simulink model "vehicle_progetto_v1_sospensioni_dual_motor"  (R2022a)
settings: Solver=ode45  StartTime=0.0  StopTime=200.0  MinStep=1e-60  RelTol=1e-3
values from neighbouring files (symbols this model uses):
  a = 1.3    [vehicle_parameters_v1_sospensioni.m]
  alpha = atan(w/(2*b))    [vehicle_parameters_v1_sospensioni.m]
  b = 1.8    [vehicle_parameters_v1_sospensioni.m]
  ca = 0.5    [vehicle_parameters_v1_sospensioni.m]
  cs = sqrt(2*ks*M)    [vehicle_parameters_v1_sospensioni.m]
  h_gc = 0.35    [vehicle_parameters_v1_sospensioni.m]
  J_motore = 0.3    [vehicle_parameters_v1_sospensioni.m]
  J_wheel = 0.4    [vehicle_parameters_v1_sospensioni.m]
  Jx = 300    [vehicle_parameters_v1_sospensioni.m]
  Jy = 500    [vehicle_parameters_v1_sospensioni.m]
  Jz = 600    [vehicle_parameters_v1_sospensioni.m]
  K_elettrica_motore = 0.1    [vehicle_parameters_v1_sospensioni.m]
  K_f_motore = 1    [vehicle_parameters_v1_sospensioni.m]
  K_motore = 1    [vehicle_parameters_v1_sospensioni.m]
  k_r = 200*1e4    (= 2000000)    [vehicle_parameters_v1_sospensioni.m]
  k_tu = 10*1.5e5    (= 1500000)    [vehicle_parameters_v1_sospensioni.m]
  k_tv = 10*40000    (= 400000)    [vehicle_parameters_v1_sospensioni.m]
  ks = 39000/4    (= 9750)    [vehicle_parameters_v1_sospensioni.m]
  L = sqrt(a^2+w^2 /4)    [vehicle_parameters_v1_sospensioni.m]
  L_motore = 0.001100    (= 0.0011)    [vehicle_parameters_v1_sospensioni.m]
  M = 1500    [vehicle_parameters_v1_sospensioni.m]
  mu_dyn = 0.2    [vehicle_parameters_v1_sospensioni.m]
  mu_st = 0.8    [vehicle_parameters_v1_sospensioni.m]
  r = 0.3    [vehicle_parameters_v1_sospensioni.m]
  R = sqrt(b^2+w^2 /4)    [vehicle_parameters_v1_sospensioni.m]
  R_motore = 0.210    (= 0.21)    [vehicle_parameters_v1_sospensioni.m]
  theta = atan(w/(2*a))    [vehicle_parameters_v1_sospensioni.m]
  w = 1.6    [vehicle_parameters_v1_sospensioni.m]
libraries: slpidlib x4, simulink x4
settings Model: Creator=jackrip  LastModifiedBy=jackrip

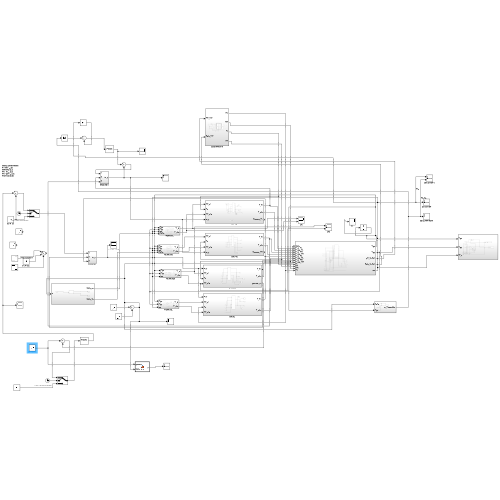
[thumbnail: Simulink's stored preview of the top-level diagram]
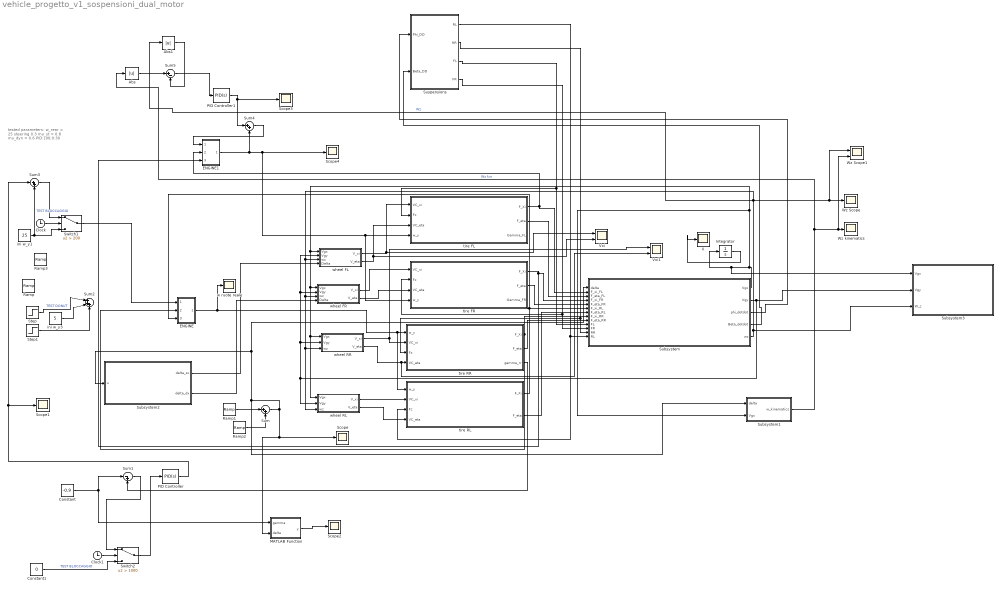
== system vehicle_progetto_v1_sospensioni_dual_motor ==
  note: tested parameters:
      | w_rear = 25
      | steering 0.3
      | mu_st = 0.8
      | mu_dyn = 0.6
      | PID:100;0;30
  Abs : Abs  SaturateOnIntegerOverflow=off
  Abs1 : Abs  SaturateOnIntegerOverflow=off
  Clock : Clock
  Clock1 : Clock
  Constant : Constant  Value=-0.9
  Constant1 : Constant  Value=0
  ENGINE : Subsystem
  ENGINE1 : Subsystem
  Integrator : Integrator
  MATLAB Function : MATLAB Function  TreatAsAtomicUnit=on
  PID Controller : slpidlib/PID Controller  Controller=PID  Form=Parallel  TimeDomain=Continuous-time  UseExternalTs=off  SampleTime=-1  IntegratorMethod=Forward Euler  FilterMethod=Forward Euler  ControllerParametersSource=internal  P=200  I=0.5  UseKiTs=off  D=0  N=100  UseFilter=on  TunerSelectOption=Transfer Function Based (PID Tuner App)  InitialConditionSource=internal  InitialConditionForIntegrator=0  InitialConditionForFilter=0  DifferentiatorICPrevScaledInput=0  ExternalReset=none  TrackingMode=off  Kt=1  LimitOutput=off  SatLimitsSource=internal  UpperSaturationLimit=inf  LowerSaturationLimit=-inf  LinearizeAsGain=on  AntiWindupMode=none  Kb=1  POutMin=[]  POutMax=[]  IOutMin=[]  IOutMax=[]  DOutMin=[]  DOutMax=[]  NOutMin=[]  NOutMax=[]  SumOutMin=[]  SumOutMax=[]  SaturationOutMin=[]  SaturationOutMax=[]  PParamMin=[]  PParamMax=[]  IParamMin=[]  IParamMax=[]  DParamMin=[]  DParamMax=[]  NParamMin=[]  NParamMax=[]  KbParamMin=[]  KbParamMax=[]  KtParamMin=[]  KtParamMax=[]  KbOutMin=[]  KbOutMax=[]  KtOutMin=[]  KtOutMax=[]  IntegratorOutMin=[]  IntegratorOutMax=[]  FilterOutMin=[]  FilterOutMax=[]  SumI1OutMin=[]  SumI1OutMax=[]  SumI2OutMin=[]  SumI2OutMax=[]  SumI3OutMin=[]  SumI3OutMax=[]  SumI4OutMin=[]  SumI4OutMax=[]  SumDOutMin=[]  SumDOutMax=[]  DifferentiatorOutMin=[]  DifferentiatorOutMax=[]  FilterDiffOutCoefMin=[]  FilterDiffOutCoefMax=[]  ReciprocalOutMin=[]  ReciprocalOutMax=[]  SumDenOutMin=[]  SumDenOutMax=[]  SumNumOutMin=[]  SumNumOutMax=[]  DivideOutMin=[]  DivideOutMax=[]  UdiffTsProdOutMin=[]  UdiffTsProdOutMax=[]  NTsProdOutMin=[]  NTsProdOutMax=[]  UintegralTsProdOutMin=[]  UintegralTsProdOutMax=[]  UngainTsProdOutMin=[]  UngainTsProdOutMax=[]  IntegratorContinuousStateAttributes=''  IntegratorStateMustResolveToSignalObject=off  IntegratorRTWStateStorageClass=Auto  FilterContinuousStateAttributes=''  FilterStateMustResolveToSignalObject=off  FilterRTWStateStorageClass=Auto  ParallelPVariant=InternalParameters  IdealPVariant=Disabled  IVariant=InternalParameters  DVariant=InternalParameters  IntegratorVariant=Continuous  SatVariant=Disabled  AWVariant=Passthrough  PCopyVariant=Disabled  TRVariant=Disabled  FdbkBlocksVariant=Forward  IdealPFdbkVariant=Disabled  SatFdbkVariant=Disabled  DerivativeFilterVariant=ContFilter  NVariant=InternalParameters  NCopyVariant=Disabled  FilterICVariant=InternalICsFilter  IntegratorICVariant=InternalICs  ExternalResetVariant=Disabled  TRSumVariant=Passthrough  SumFdbkVariant=Disabled  SumVariant=Sum_PID  TsampFilterVariant=InternalTs  TsampNgainVariant=Passthrough  TsampIntegralVariant=Passthrough  ExternalSaturationOutDataTypeStr=Inherit: Same as second input  aMode=0
  PID Controller1 : slpidlib/PID Controller  Controller=PID  Form=Parallel  TimeDomain=Continuous-time  UseExternalTs=off  SampleTime=-1  IntegratorMethod=Forward Euler  FilterMethod=Forward Euler  ControllerParametersSource=internal  P=100  I=0  UseKiTs=off  D=30  N=100  UseFilter=on  TunerSelectOption=Transfer Function Based (PID Tuner App)  InitialConditionSource=internal  InitialConditionForIntegrator=0  InitialConditionForFilter=0  DifferentiatorICPrevScaledInput=0  ExternalReset=none  TrackingMode=off  Kt=1  LimitOutput=off  SatLimitsSource=internal  UpperSaturationLimit=inf  LowerSaturationLimit=-inf  LinearizeAsGain=on  AntiWindupMode=none  Kb=1  POutMin=[]  POutMax=[]  IOutMin=[]  IOutMax=[]  DOutMin=[]  DOutMax=[]  NOutMin=[]  NOutMax=[]  SumOutMin=[]  SumOutMax=[]  SaturationOutMin=[]  SaturationOutMax=[]  PParamMin=[]  PParamMax=[]  IParamMin=[]  IParamMax=[]  DParamMin=[]  DParamMax=[]  NParamMin=[]  NParamMax=[]  KbParamMin=[]  KbParamMax=[]  KtParamMin=[]  KtParamMax=[]  KbOutMin=[]  KbOutMax=[]  KtOutMin=[]  KtOutMax=[]  IntegratorOutMin=[]  IntegratorOutMax=[]  FilterOutMin=[]  FilterOutMax=[]  SumI1OutMin=[]  SumI1OutMax=[]  SumI2OutMin=[]  SumI2OutMax=[]  SumI3OutMin=[]  SumI3OutMax=[]  SumI4OutMin=[]  SumI4OutMax=[]  SumDOutMin=[]  SumDOutMax=[]  DifferentiatorOutMin=[]  DifferentiatorOutMax=[]  FilterDiffOutCoefMin=[]  FilterDiffOutCoefMax=[]  ReciprocalOutMin=[]  ReciprocalOutMax=[]  SumDenOutMin=[]  SumDenOutMax=[]  SumNumOutMin=[]  SumNumOutMax=[]  DivideOutMin=[]  DivideOutMax=[]  UdiffTsProdOutMin=[]  UdiffTsProdOutMax=[]  NTsProdOutMin=[]  NTsProdOutMax=[]  UintegralTsProdOutMin=[]  UintegralTsProdOutMax=[]  UngainTsProdOutMin=[]  UngainTsProdOutMax=[]  IntegratorContinuousStateAttributes=''  IntegratorStateMustResolveToSignalObject=off  IntegratorRTWStateStorageClass=Auto  FilterContinuousStateAttributes=''  FilterStateMustResolveToSignalObject=off  FilterRTWStateStorageClass=Auto  ParallelPVariant=InternalParameters  IdealPVariant=Disabled  IVariant=InternalParameters  DVariant=InternalParameters  IntegratorVariant=Continuous  SatVariant=Disabled  AWVariant=Passthrough  PCopyVariant=Disabled  TRVariant=Disabled  FdbkBlocksVariant=Forward  IdealPFdbkVariant=Disabled  SatFdbkVariant=Disabled  DerivativeFilterVariant=ContFilter  NVariant=InternalParameters  NCopyVariant=Disabled  FilterICVariant=InternalICsFilter  IntegratorICVariant=InternalICs  ExternalResetVariant=Disabled  TRSumVariant=Passthrough  SumFdbkVariant=Disabled  SumVariant=Sum_PID  TsampFilterVariant=InternalTs  TsampNgainVariant=Passthrough  TsampIntegralVariant=Passthrough  ExternalSaturationOutDataTypeStr=Inherit: Same as second input  aMode=0
  Ramp : simulink/Sources/Ramp  slope=0  start=100  InitialOutput=0
  Ramp1 : simulink/Sources/Ramp  slope=0.3  start=50  InitialOutput=0
  Ramp2 : simulink/Sources/Ramp  slope=-0.3  start=50.5  InitialOutput=0
  Ramp3 : simulink/Sources/Ramp  slope=0  start=103  InitialOutput=0
  Scope{,1..4} (5 alike) : Scope
  Step : Step  Time=100  After=25  SampleTime=0
  Step1 : Step  Time=101.5  After=-25  SampleTime=0
  Subsystem : Subsystem
  Subsystem1 : Subsystem
  Subsystem2 : Subsystem
  Subsystem3 : Subsystem
  Sum : Sum  Inputs=|++
  Sum1 : Sum  Inputs=|-+
  Sum2 : Sum  Inputs=|+++
  Sum3 : Sum  Inputs=|++
  Sum4 : Sum  Inputs=|++
  Sum5 : Sum  Inputs=|+-
  Suspensions : Subsystem
  Switch1 : Switch  Criteria=u2 > Threshold  Threshold=200  SaturateOnIntegerOverflow=off  InputSameDT=off
  Switch2 : Switch  Criteria=u2 > Threshold  Threshold=1000  SaturateOnIntegerOverflow=off  InputSameDT=off
  Vxi : Scope  NumInputPorts=2
  Vxi1 : Scope  NumInputPorts=2
  Wz Scope : Scope
  Wz Scope1 : Scope  NumInputPorts=2
  Wz kinematics : Scope
  X : Scope
  ini w_y1 : Constant  Value=25
  ini w_y3 : Constant  Value=5
  tire FL : Subsystem
  tire FR : Subsystem
  tire RL : Subsystem
  tire RR : Subsystem
  w ruote reale : Scope
  wheel FL : Subsystem
  wheel FR : Subsystem
  wheel RL : Subsystem
  wheel RR : Subsystem
  wires:
  wheel FL/1(V_xi) -> Vxi/1, tire FL/1(VC_xi)
  wheel FL/2(V_eta) -> Vxi/2, tire FL/3(VC_eta)
  tire FL/1(F_Xi) -> Subsystem/2(F_xi_FL), ENGINE1/2(Input1)
  tire FL/2(F_eta) -> Subsystem/3(F_eta_FL)
  tire RL/1(F_Xi) -> ENGINE/3(Input2), Subsystem/6(F_xi_RL)
  tire RL/2(F_eta) -> Subsystem/7(F_eta_RL)
  tire RR/1(F_Xi) -> ENGINE/2(Input1), Subsystem/8(F_xi_RR)
  tire RR/2(F_eta) -> Subsystem/9(F_eta_RR)
  tire FR/1(F_Xi) -> ENGINE1/3(Input2), Subsystem/4(F_xi_FR)
  tire FR/2(F_eta) -> Subsystem/5(F_eta_FR)
  wheel FR/1(V_xi) -> tire FR/1(VC_xi)
  wheel FR/2(V_eta) -> tire FR/3(VC_eta)
  wheel RL/1(V_xi) -> tire RL/2(VC_xi)
  wheel RR/1(V_xi) -> Vxi1/1, tire RR/2(VC_xi)
  wheel RR/2(V_eta) -> Vxi1/2, tire RR/4(VC_eta)
  wheel RL/2(V_eta) -> tire RL/4(VC_eta)
  Subsystem/1(Vgx) -> wheel RL/1(Vgx), wheel RR/1(Vgx), wheel FR/1(Vgx), wheel FL/1(Vgx), Subsystem1/2(Vgx), Subsystem3/1(Vgx), Integrator/1
  Subsystem/2(Vgy) -> Subsystem3/2(Vgy), wheel FL/2(Vgy), wheel FR/2(Vgy), wheel RR/2(Vgy), wheel RL/2(Vgy)
  Subsystem/5(wz) -> Subsystem3/3(W_z), Abs1/1, Wz Scope1/1, Wz Scope/1, wheel RL/3(wz), wheel RR/3(wz), wheel FR/3(wz), wheel FL/3(wz)  "Wz"
  Ramp2/1 -> Sum/2
  Ramp1/1 -> Sum/1
  Integrator/1 -> X/1
  Clock/1 -> Switch1/2
  ini w_y1/1 -> Switch1/3, Sum3/2  "TEST BLOCCAGGIO"
  ini w_y3/1 -> Sum2/2
  Sum/1 -> MATLAB Function/2(delta), Scope/1, Subsystem2/1(u), Subsystem/1(delta), Subsystem1/1(delta)
  Step/1 -> Sum2/1  "TEST DONUT"
  Step1/1 -> Sum2/3
  Subsystem1/1(w_kinematics) -> Abs/1, Wz Scope1/2, Wz kinematics/1  "Wz kin"
  Subsystem2/1(delta_sx) -> wheel FL/4(Delta)
  Subsystem2/2(delta_dx) -> wheel FR/4(Delta)
  ENGINE/1(w_y) -> w ruote reale/1, tire RR/1(w_y), tire RL/1(w_y)
  Suspensions/3(FL) -> Subsystem/10(FL), tire FL/2(Fz)
  Suspensions/4(FR) -> tire FR/2(Fz), Subsystem/11(FR)
  Suspensions/2(RR) -> Subsystem/12(RR), tire RR/3(Fz)
  Suspensions/1(RL) -> tire RL/3(Fz), Subsystem/13(RL)
  Subsystem/3(phi_dotdot) -> Suspensions/1(Phi_DD)
  Subsystem/4(Beta_dotdot) -> Suspensions/2(Beta_DD)
  Constant/1 -> MATLAB Function/1(gamma), Sum1/1
  tire RR/3(gamma_rr) -> Sum1/2
  Switch1/1 -> ENGINE/1(Input)
  PID Controller/1 -> Scope1/1, Sum3/1
  Sum3/1 -> Switch1/1
  Clock1/1 -> Switch2/2
  Constant1/1 -> Switch2/3  "TEST BLOCCAGGIO"
  Sum1/1 -> Switch2/1
  Switch2/1 -> PID Controller/1
  MATLAB Function/1(y) -> Scope2/1
  ENGINE1/1(w_y) -> Sum4/2, tire FR/4(w_y), tire FL/4(w_y), Scope4/1
  Sum4/1 -> ENGINE1/1(Input)
  PID Controller1/1 -> Sum4/1, Scope3/1
  Abs/1 -> Sum5/1
  Abs1/1 -> Sum5/2
  Sum5/1 -> PID Controller1/1

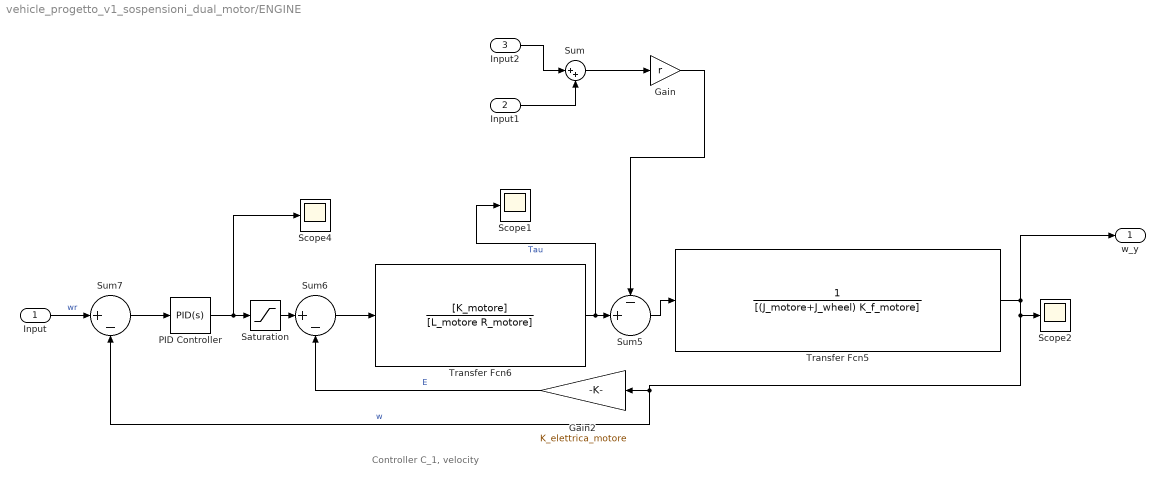
== system vehicle_progetto_v1_sospensioni_dual_motor/ENGINE ==
  note: Controller C_1, velocity
  Input : Inport
  Input1 : Inport  Port=2
  Input2 : Inport  Port=3
  Gain : Gain  Gain=r
  Gain2 : Gain  Gain=K_elettrica_motore
  PID Controller : slpidlib/PID Controller  Controller=PID  Form=Parallel  TimeDomain=Continuous-time  UseExternalTs=off  SampleTime=-1  IntegratorMethod=Forward Euler  FilterMethod=Forward Euler  ControllerParametersSource=internal  P=8  I=0.5  UseKiTs=off  D=0.1  N=100  UseFilter=on  TunerSelectOption=Transfer Function Based (PID Tuner App)  InitialConditionSource=internal  InitialConditionForIntegrator=0  InitialConditionForFilter=0  DifferentiatorICPrevScaledInput=0  ExternalReset=none  TrackingMode=off  Kt=1  LimitOutput=off  SatLimitsSource=internal  UpperSaturationLimit=inf  LowerSaturationLimit=-inf  LinearizeAsGain=on  AntiWindupMode=none  Kb=1  POutMin=[]  POutMax=[]  IOutMin=[]  IOutMax=[]  DOutMin=[]  DOutMax=[]  NOutMin=[]  NOutMax=[]  SumOutMin=[]  SumOutMax=[]  SaturationOutMin=[]  SaturationOutMax=[]  PParamMin=[]  PParamMax=[]  IParamMin=[]  IParamMax=[]  DParamMin=[]  DParamMax=[]  NParamMin=[]  NParamMax=[]  KbParamMin=[]  KbParamMax=[]  KtParamMin=[]  KtParamMax=[]  KbOutMin=[]  KbOutMax=[]  KtOutMin=[]  KtOutMax=[]  IntegratorOutMin=[]  IntegratorOutMax=[]  FilterOutMin=[]  FilterOutMax=[]  SumI1OutMin=[]  SumI1OutMax=[]  SumI2OutMin=[]  SumI2OutMax=[]  SumI3OutMin=[]  SumI3OutMax=[]  SumI4OutMin=[]  SumI4OutMax=[]  SumDOutMin=[]  SumDOutMax=[]  DifferentiatorOutMin=[]  DifferentiatorOutMax=[]  FilterDiffOutCoefMin=[]  FilterDiffOutCoefMax=[]  ReciprocalOutMin=[]  ReciprocalOutMax=[]  SumDenOutMin=[]  SumDenOutMax=[]  SumNumOutMin=[]  SumNumOutMax=[]  DivideOutMin=[]  DivideOutMax=[]  UdiffTsProdOutMin=[]  UdiffTsProdOutMax=[]  NTsProdOutMin=[]  NTsProdOutMax=[]  UintegralTsProdOutMin=[]  UintegralTsProdOutMax=[]  UngainTsProdOutMin=[]  UngainTsProdOutMax=[]  IntegratorContinuousStateAttributes=''  IntegratorStateMustResolveToSignalObject=off  IntegratorRTWStateStorageClass=Auto  FilterContinuousStateAttributes=''  FilterStateMustResolveToSignalObject=off  FilterRTWStateStorageClass=Auto  ParallelPVariant=InternalParameters  IdealPVariant=Disabled  IVariant=InternalParameters  DVariant=InternalParameters  IntegratorVariant=Continuous  SatVariant=Disabled  AWVariant=Passthrough  PCopyVariant=Disabled  TRVariant=Disabled  FdbkBlocksVariant=Forward  IdealPFdbkVariant=Disabled  SatFdbkVariant=Disabled  DerivativeFilterVariant=ContFilter  NVariant=InternalParameters  NCopyVariant=Disabled  FilterICVariant=InternalICsFilter  IntegratorICVariant=InternalICs  ExternalResetVariant=Disabled  TRSumVariant=Passthrough  SumFdbkVariant=Disabled  SumVariant=Sum_PID  TsampFilterVariant=InternalTs  TsampNgainVariant=Passthrough  TsampIntegralVariant=Passthrough  ExternalSaturationOutDataTypeStr=Inherit: Same as second input  aMode=0
  Saturation : Saturate  UpperLimit=400  LowerLimit=-1000
  Scope1 : Scope
  Scope2 : Scope
  Scope4 : Scope
  Sum : Sum  Inputs=|++
  Sum5 : Sum  Inputs=-+|
  Sum6 : Sum  Inputs=|+-
  Sum7 : Sum  Inputs=|+-
  Transfer Fcn5 : TransferFcn  Denominator=[(J_motore+J_wheel) K_f_motore]
  Transfer Fcn6 : TransferFcn  Numerator=[K_motore]  Denominator=[L_motore R_motore]
  w_y : Outport
  wires:
  Sum7/1 -> PID Controller/1
  Sum5/1 -> Transfer Fcn5/1
  Gain/1 -> Sum5/1
  Gain2/1 -> Sum6/2  "E"
  Sum6/1 -> Transfer Fcn6/1
  Transfer Fcn6/1 -> Scope1/1, Sum5/2  "Tau"
  Input/1 -> Sum7/1  "wr"
  PID Controller/1 -> Scope4/1, Saturation/1
  Transfer Fcn5/1 -> w_y/1, Gain2/1, Sum7/2, Scope2/1  "w"
  Input2/1 -> Sum/1
  Input1/1 -> Sum/2
  Sum/1 -> Gain/1
  Saturation/1 -> Sum6/1

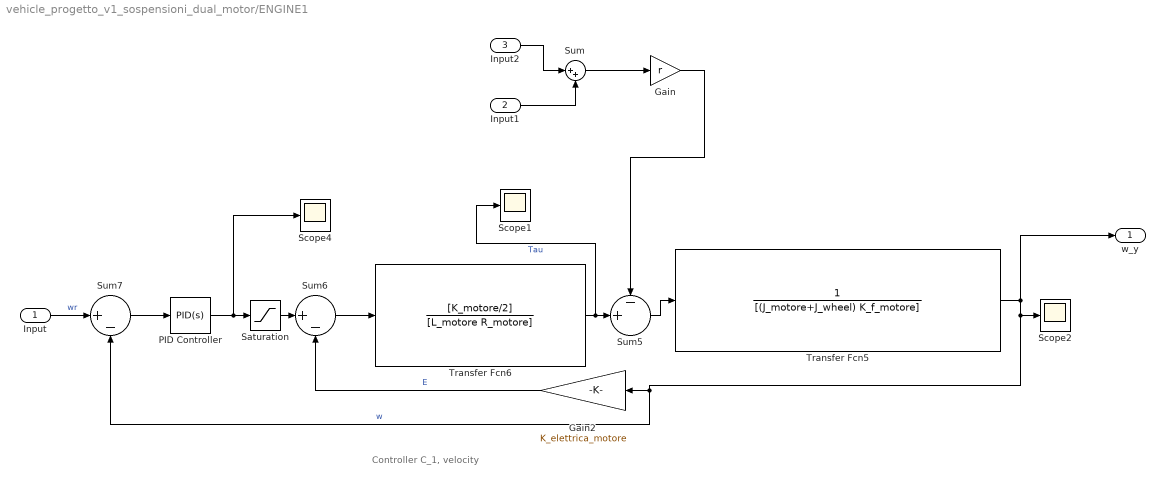
== system vehicle_progetto_v1_sospensioni_dual_motor/ENGINE1 ==
  note: Controller C_1, velocity
  Input : Inport
  Input1 : Inport  Port=2
  Input2 : Inport  Port=3
  Gain : Gain  Gain=r
  Gain2 : Gain  Gain=K_elettrica_motore
  PID Controller : slpidlib/PID Controller  Controller=PID  Form=Parallel  TimeDomain=Continuous-time  UseExternalTs=off  SampleTime=-1  IntegratorMethod=Forward Euler  FilterMethod=Forward Euler  ControllerParametersSource=internal  P=8  I=0.5  UseKiTs=off  D=0.1  N=100  UseFilter=on  TunerSelectOption=Transfer Function Based (PID Tuner App)  InitialConditionSource=internal  InitialConditionForIntegrator=0  InitialConditionForFilter=0  DifferentiatorICPrevScaledInput=0  ExternalReset=none  TrackingMode=off  Kt=1  LimitOutput=off  SatLimitsSource=internal  UpperSaturationLimit=inf  LowerSaturationLimit=-inf  LinearizeAsGain=on  AntiWindupMode=none  Kb=1  POutMin=[]  POutMax=[]  IOutMin=[]  IOutMax=[]  DOutMin=[]  DOutMax=[]  NOutMin=[]  NOutMax=[]  SumOutMin=[]  SumOutMax=[]  SaturationOutMin=[]  SaturationOutMax=[]  PParamMin=[]  PParamMax=[]  IParamMin=[]  IParamMax=[]  DParamMin=[]  DParamMax=[]  NParamMin=[]  NParamMax=[]  KbParamMin=[]  KbParamMax=[]  KtParamMin=[]  KtParamMax=[]  KbOutMin=[]  KbOutMax=[]  KtOutMin=[]  KtOutMax=[]  IntegratorOutMin=[]  IntegratorOutMax=[]  FilterOutMin=[]  FilterOutMax=[]  SumI1OutMin=[]  SumI1OutMax=[]  SumI2OutMin=[]  SumI2OutMax=[]  SumI3OutMin=[]  SumI3OutMax=[]  SumI4OutMin=[]  SumI4OutMax=[]  SumDOutMin=[]  SumDOutMax=[]  DifferentiatorOutMin=[]  DifferentiatorOutMax=[]  FilterDiffOutCoefMin=[]  FilterDiffOutCoefMax=[]  ReciprocalOutMin=[]  ReciprocalOutMax=[]  SumDenOutMin=[]  SumDenOutMax=[]  SumNumOutMin=[]  SumNumOutMax=[]  DivideOutMin=[]  DivideOutMax=[]  UdiffTsProdOutMin=[]  UdiffTsProdOutMax=[]  NTsProdOutMin=[]  NTsProdOutMax=[]  UintegralTsProdOutMin=[]  UintegralTsProdOutMax=[]  UngainTsProdOutMin=[]  UngainTsProdOutMax=[]  IntegratorContinuousStateAttributes=''  IntegratorStateMustResolveToSignalObject=off  IntegratorRTWStateStorageClass=Auto  FilterContinuousStateAttributes=''  FilterStateMustResolveToSignalObject=off  FilterRTWStateStorageClass=Auto  ParallelPVariant=InternalParameters  IdealPVariant=Disabled  IVariant=InternalParameters  DVariant=InternalParameters  IntegratorVariant=Continuous  SatVariant=Disabled  AWVariant=Passthrough  PCopyVariant=Disabled  TRVariant=Disabled  FdbkBlocksVariant=Forward  IdealPFdbkVariant=Disabled  SatFdbkVariant=Disabled  DerivativeFilterVariant=ContFilter  NVariant=InternalParameters  NCopyVariant=Disabled  FilterICVariant=InternalICsFilter  IntegratorICVariant=InternalICs  ExternalResetVariant=Disabled  TRSumVariant=Passthrough  SumFdbkVariant=Disabled  SumVariant=Sum_PID  TsampFilterVariant=InternalTs  TsampNgainVariant=Passthrough  TsampIntegralVariant=Passthrough  ExternalSaturationOutDataTypeStr=Inherit: Same as second input  aMode=0
  Saturation : Saturate  UpperLimit=400  LowerLimit=-1000
  Scope1 : Scope
  Scope2 : Scope
  Scope4 : Scope
  Sum : Sum  Inputs=|++
  Sum5 : Sum  Inputs=-+|
  Sum6 : Sum  Inputs=|+-
  Sum7 : Sum  Inputs=|+-
  Transfer Fcn5 : TransferFcn  Denominator=[(J_motore+J_wheel) K_f_motore]
  Transfer Fcn6 : TransferFcn  Numerator=[K_motore/2]  Denominator=[L_motore R_motore]
  w_y : Outport
  wires:
  Sum7/1 -> PID Controller/1
  Sum5/1 -> Transfer Fcn5/1
  Gain/1 -> Sum5/1
  Gain2/1 -> Sum6/2  "E"
  Sum6/1 -> Transfer Fcn6/1
  Transfer Fcn6/1 -> Scope1/1, Sum5/2  "Tau"
  Input/1 -> Sum7/1  "wr"
  PID Controller/1 -> Scope4/1, Saturation/1
  Transfer Fcn5/1 -> w_y/1, Gain2/1, Sum7/2, Scope2/1  "w"
  Input2/1 -> Sum/1
  Input1/1 -> Sum/2
  Sum/1 -> Gain/1
  Saturation/1 -> Sum6/1

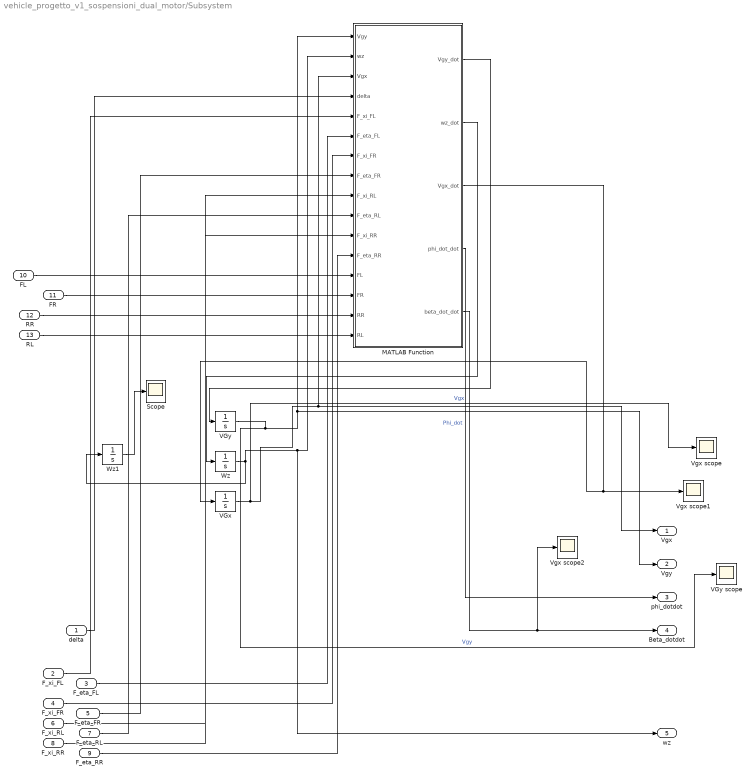
== system vehicle_progetto_v1_sospensioni_dual_motor/Subsystem ==
  delta : Inport
  F_xi_FL : Inport  Port=2
  F_eta_FL : Inport  Port=3
  F_xi_FR : Inport  Port=4
  F_eta_FR : Inport  Port=5
  F_xi_RL : Inport  Port=6
  F_eta_RL : Inport  Port=7
  F_xi_RR : Inport  Port=8
  F_eta_RR : Inport  Port=9
  FL : Inport  Port=10
  FR : Inport  Port=11
  RR : Inport  Port=12
  RL : Inport  Port=13
  " VGy scope" : Scope
  MATLAB Function : MATLAB Function  TreatAsAtomicUnit=on
  Scope : Scope
  VGx : Integrator  InitialCondition=0.055
  VGy : Integrator
  Vgx scope : Scope
  Vgx scope1 : Scope
  Vgx scope2 : Scope
  Wz : Integrator
  Wz1 : Integrator
  Vgx : Outport
  Vgy : Outport  Port=2
  phi_dotdot : Outport  Port=3
  Beta_dotdot : Outport  Port=4
  wz : Outport  Port=5
  wires:
  MATLAB Function/4(phi_dot_dot) -> phi_dotdot/1  "Phi_dot"
  VGy/1 -> Vgy/1, MATLAB Function/1(Vgy), " VGy scope"/1  "Vgy"
  MATLAB Function/2(wz_dot) -> Wz/1
  Wz/1 -> Wz1/1, wz/1, MATLAB Function/2(wz)
  MATLAB Function/3(Vgx_dot) -> VGx/1, Vgx scope1/1
  VGx/1 -> Vgx scope/1, Vgx/1, MATLAB Function/3(Vgx)  "Vgx"
  MATLAB Function/5(beta_dot_dot) -> Vgx scope2/1, Beta_dotdot/1
  delta/1 -> MATLAB Function/4(delta)
  F_xi_FL/1 -> MATLAB Function/5(F_xi_FL)
  F_eta_FL/1 -> MATLAB Function/6(F_eta_FL)
  F_xi_FR/1 -> MATLAB Function/7(F_xi_FR)
  F_eta_FR/1 -> MATLAB Function/8(F_eta_FR)
  F_xi_RL/1 -> MATLAB Function/9(F_xi_RL)
  F_eta_RL/1 -> MATLAB Function/10(F_eta_RL)
  F_xi_RR/1 -> MATLAB Function/11(F_xi_RR)
  F_eta_RR/1 -> MATLAB Function/12(F_eta_RR)
  Wz1/1 -> Scope/1
  MATLAB Function/1(Vgy_dot) -> VGy/1
  RL/1 -> MATLAB Function/16(RL)
  RR/1 -> MATLAB Function/15(RR)
  FR/1 -> MATLAB Function/14(FR)
  FL/1 -> MATLAB Function/13(FL)

== system vehicle_progetto_v1_sospensioni_dual_motor/Subsystem1 ==
  delta : Inport
  Vgx : Inport  Port=2
  MATLAB Function : MATLAB Function  TreatAsAtomicUnit=on
  w_kinematics : Outport
  wires:
  Vgx/1 -> MATLAB Function/2(vgx)
  delta/1 -> MATLAB Function/1(delta)
  MATLAB Function/1(w_kinematics) -> w_kinematics/1

== system vehicle_progetto_v1_sospensioni_dual_motor/Subsystem2 ==
  u : Inport
  MATLAB Function : MATLAB Function  TreatAsAtomicUnit=on
  delta_sx : Outport
  delta_dx : Outport  Port=2
  wires:
  u/1 -> MATLAB Function/1(u)
  MATLAB Function/1(delta_sx) -> delta_sx/1
  MATLAB Function/2(delta_dx) -> delta_dx/1

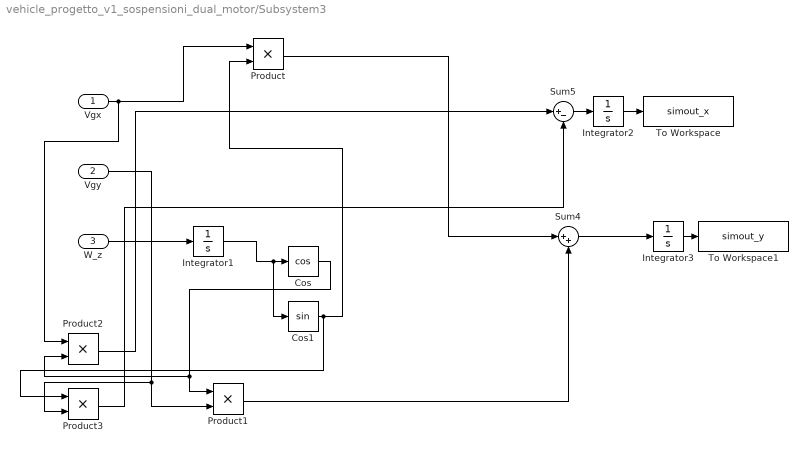
== system vehicle_progetto_v1_sospensioni_dual_motor/Subsystem3 ==
  Vgx : Inport
  Vgy : Inport  Port=2
  W_z : Inport  Port=3
  Cos : Trigonometry  Operator=cos
  Cos1 : Trigonometry
  Integrator1 : Integrator
  Integrator2 : Integrator
  Integrator3 : Integrator
  Product{,1..3} (4 alike) : Product
  Sum4 : Sum  Inputs=|++
  Sum5 : Sum  Inputs=|+-
  To Workspace : ToWorkspace  VariableName=simout_x  SaveFormat=Timeseries  SampleTime=-1
  To Workspace1 : ToWorkspace  VariableName=simout_y  SaveFormat=Timeseries  SampleTime=-1
  wires:
  Integrator2/1 -> To Workspace/1
  Integrator3/1 -> To Workspace1/1
  Product2/1 -> Sum5/1
  Sum4/1 -> Integrator3/1
  Product1/1 -> Sum4/2
  Product/1 -> Sum4/1
  W_z/1 -> Integrator1/1
  Product3/1 -> Sum5/2
  Cos1/1 -> Product3/1, Product/2
  Vgy/1 -> Product1/2, Product3/2
  Vgx/1 -> Product2/1, Product/1
  Integrator1/1 -> Cos1/1, Cos/1
  Cos/1 -> Product2/2, Product1/1
  Sum5/1 -> Integrator2/1

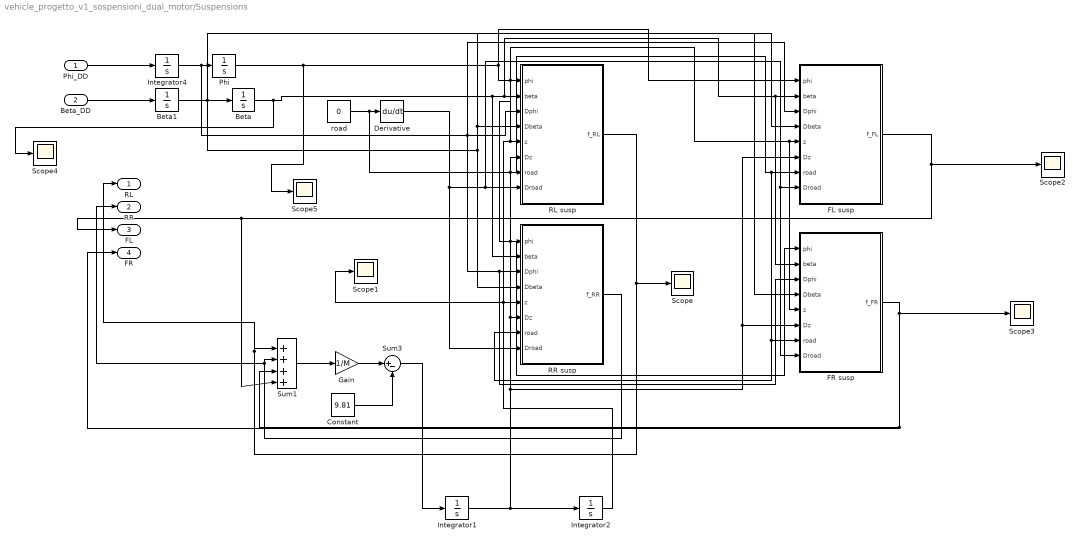
== system vehicle_progetto_v1_sospensioni_dual_motor/Suspensions ==
  Phi_DD : Inport
  Beta_DD : Inport  Port=2
  Beta : Integrator
  Beta1 : Integrator
  Constant : Constant  Value=9.81
  Derivative : Derivative
  FL susp : MATLAB Function  TreatAsAtomicUnit=on
  FR susp : MATLAB Function  TreatAsAtomicUnit=on
  Gain : Gain  Gain=1/M
  Integrator1 : Integrator
  Integrator2 : Integrator  InitialCondition=-0.377
  Integrator4 : Integrator
  Phi : Integrator
  RL susp : MATLAB Function  TreatAsAtomicUnit=on
  RR susp : MATLAB Function  TreatAsAtomicUnit=on
  Scope{,1..5} (6 alike) : Scope
  Sum1 : Sum  Inputs=|++++
  Sum3 : Sum  Inputs=|+-
  road : Constant  Value=0
  RL : Outport
  RR : Outport  Port=2
  FL : Outport  Port=3
  FR : Outport  Port=4
  wires:
  Phi_DD/1 -> Integrator4/1
  RL susp/1(f_RL) -> Scope/1, RL/1, Sum1/1
  Integrator4/1 -> RL susp/3(Dphi), RR susp/3(Dphi), FR susp/3(Dphi), FL susp/3(Dphi), Phi/1
  Sum3/1 -> Integrator1/1
  Sum1/1 -> Gain/1
  FL susp/1(f_FL) -> Scope2/1, FL/1, Sum1/4
  Gain/1 -> Sum3/1
  Integrator1/1 -> RL susp/6(Dz), RR susp/6(Dz), FR susp/6(Dz), FL susp/6(Dz), Integrator2/1
  Beta1/1 -> Beta/1, RR susp/4(Dbeta), RL susp/4(Dbeta), FL susp/4(Dbeta), FR susp/4(Dbeta)
  Derivative/1 -> RL susp/8(Droad), FL susp/8(Droad), FR susp/8(Droad), RR susp/8(Droad)
  Integrator2/1 -> Scope1/1, RR susp/5(z), FR susp/5(z), FL susp/5(z), RL susp/5(z)
  Constant/1 -> Sum3/2
  FR susp/1(f_FR) -> FR/1, Sum1/3, Scope3/1
  RR susp/1(f_RR) -> RR/1, Sum1/2
  Beta_DD/1 -> Beta1/1
  Phi/1 -> Scope5/1, FR susp/1(phi), RR susp/1(phi), RL susp/1(phi), FL susp/1(phi)
  road/1 -> FL susp/7(road), RR susp/7(road), FR susp/7(road), RL susp/7(road), Derivative/1
  Beta/1 -> Scope4/1, FL susp/2(beta), FR susp/2(beta), RL susp/2(beta), RR susp/2(beta)

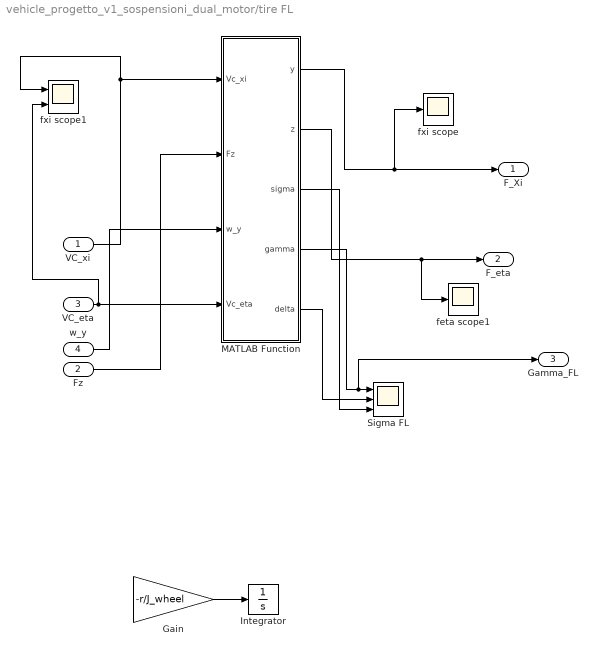
== system vehicle_progetto_v1_sospensioni_dual_motor/tire FL ==
  VC_xi : Inport
  Fz : Inport  Port=2
  VC_eta : Inport  Port=3
  w_y : Inport  Port=4
  Gain : Gain  Gain=-r/J_wheel
  Integrator : Integrator  InitialCondition=0.0001
  MATLAB Function : MATLAB Function  TreatAsAtomicUnit=on
  Sigma FL : Scope  NumInputPorts=3
  feta scope1 : Scope
  fxi scope : Scope
  fxi scope1 : Scope  NumInputPorts=2
  F_Xi : Outport
  F_eta : Outport  Port=2
  Gamma_FL : Outport  Port=3
  wires:
  MATLAB Function/1(y) -> F_Xi/1, fxi scope/1
  MATLAB Function/2(z) -> feta scope1/1, F_eta/1
  VC_eta/1 -> fxi scope1/2, MATLAB Function/4(Vc_eta)
  MATLAB Function/3(sigma) -> Sigma FL/3
  MATLAB Function/4(gamma) -> Gamma_FL/1, Sigma FL/1
  MATLAB Function/5(delta) -> Sigma FL/2
  Gain/1 -> Integrator/1
  VC_xi/1 -> fxi scope1/1, MATLAB Function/1(Vc_xi)
  Fz/1 -> MATLAB Function/2(Fz)
  w_y/1 -> MATLAB Function/3(w_y)

== system vehicle_progetto_v1_sospensioni_dual_motor/tire FR ==
  VC_xi : Inport
  Fz : Inport  Port=2
  VC_eta : Inport  Port=3
  w_y : Inport  Port=4
  MATLAB Function : MATLAB Function  TreatAsAtomicUnit=on
  Scope : Scope
  Scope1 : Scope  NumInputPorts=2
  F_Xi : Outport
  F_eta : Outport  Port=2
  Gamma_FR : Outport  Port=3
  wires:
  MATLAB Function/1(y) -> F_Xi/1
  VC_xi/1 -> MATLAB Function/1(Vc_xi)
  MATLAB Function/2(z) -> Scope/1, F_eta/1
  VC_eta/1 -> MATLAB Function/4(Vc_eta)
  MATLAB Function/3(delta) -> Scope1/1
  MATLAB Function/4(gamma) -> Scope1/2, Gamma_FR/1
  Fz/1 -> MATLAB Function/2(Fz)
  w_y/1 -> MATLAB Function/3(w_y)

== system vehicle_progetto_v1_sospensioni_dual_motor/tire RL ==
  w_y : Inport
  VC_xi : Inport  Port=2
      settings: AttributesFormatString=|
      | Velocità Del centro della ruota diretta lungo l'asse della ruota
      | Se la macchina stesse andando dritta sarebbe uguale a vgx
  Fz : Inport  Port=3
  VC_eta : Inport  Port=4
  MATLAB Function : MATLAB Function  TreatAsAtomicUnit=on
  Scope : Scope
  Scope1 : Scope
  Scope2 : Scope
  F_Xi : Outport
  F_eta : Outport  Port=2
  wires:
  MATLAB Function/1(y) -> Scope2/1, F_Xi/1
  VC_xi/1 -> MATLAB Function/1(Vc_xi)
  w_y/1 -> MATLAB Function/3(w_y)
  MATLAB Function/2(z) -> Scope/1, Scope1/1, F_eta/1
  VC_eta/1 -> MATLAB Function/4(Vc_eta)
  Fz/1 -> MATLAB Function/2(Fz)

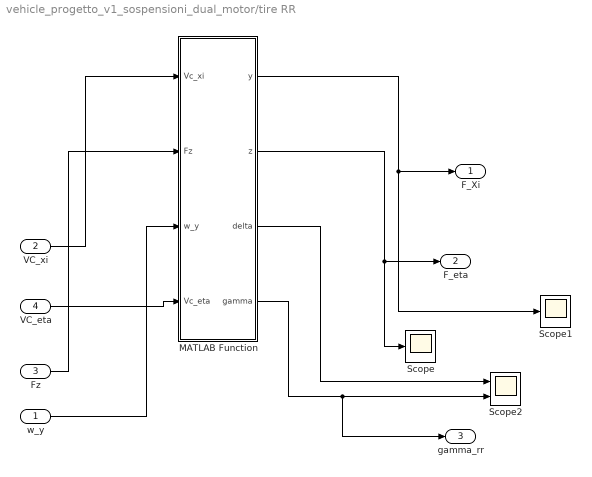
== system vehicle_progetto_v1_sospensioni_dual_motor/tire RR ==
  w_y : Inport
  VC_xi : Inport  Port=2
  Fz : Inport  Port=3
  VC_eta : Inport  Port=4
  MATLAB Function : MATLAB Function  TreatAsAtomicUnit=on
  Scope : Scope
  Scope1 : Scope
  Scope2 : Scope  NumInputPorts=2
  F_Xi : Outport
  F_eta : Outport  Port=2
  gamma_rr : Outport  Port=3
  wires:
  MATLAB Function/1(y) -> Scope1/1, F_Xi/1
  VC_xi/1 -> MATLAB Function/1(Vc_xi)
  w_y/1 -> MATLAB Function/3(w_y)
  MATLAB Function/2(z) -> Scope/1, F_eta/1
  VC_eta/1 -> MATLAB Function/4(Vc_eta)
  MATLAB Function/3(delta) -> Scope2/1
  MATLAB Function/4(gamma) -> gamma_rr/1, Scope2/2
  Fz/1 -> MATLAB Function/2(Fz)

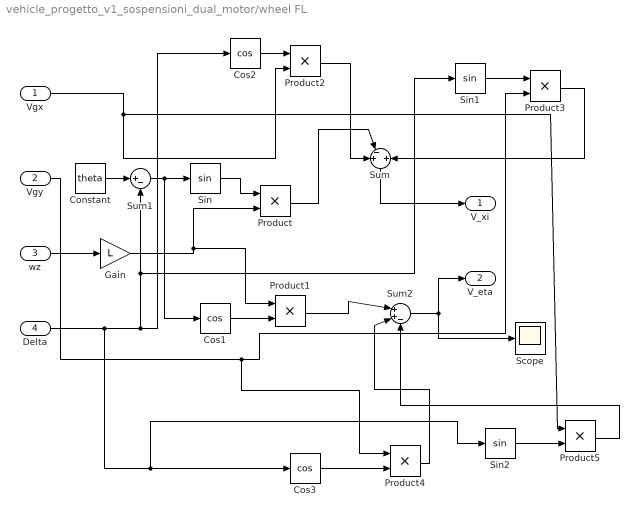
== system vehicle_progetto_v1_sospensioni_dual_motor/wheel FL ==
  Vgx : Inport
  Vgy : Inport  Port=2
  wz : Inport  Port=3
  Delta : Inport  Port=4
  Constant : Constant  Value=theta
  Cos1 : Trigonometry  Operator=cos
  Cos2 : Trigonometry  Operator=cos
  Cos3 : Trigonometry  Operator=cos
  Gain : Gain  Gain=L
  Product{,1..5} (6 alike) : Product
  Scope : Scope
  Sin : Trigonometry
  Sin1 : Trigonometry
  Sin2 : Trigonometry
  Sum : Sum  Inputs=+-|+
  Sum1 : Sum  Inputs=|+-
  Sum2 : Sum  Inputs=|++-
  V_xi : Outport
  V_eta : Outport  Port=2
  wires:
  Vgx/1 -> Product5/1, Product2/2
  wz/1 -> Gain/1
  Sin/1 -> Product/1
  Constant/1 -> Sum1/1
  Sum1/1 -> Cos1/1, Sin/1
  Delta/1 -> Sin2/1, Cos3/1, Sum1/2, Sin1/1, Cos2/1
  Product/1 -> Sum/2
  Sum/1 -> V_xi/1
  Cos1/1 -> Product1/2
  Gain/1 -> Product/2, Product1/1
  Product1/1 -> Sum2/1
  Sum2/1 -> Scope/1, V_eta/1
  Vgy/1 -> Product4/1, Product3/2
  Cos2/1 -> Product2/1
  Product2/1 -> Sum/1
  Sin1/1 -> Product3/1
  Product3/1 -> Sum/3
  Cos3/1 -> Product4/2
  Product4/1 -> Sum2/2
  Sin2/1 -> Product5/2
  Product5/1 -> Sum2/3

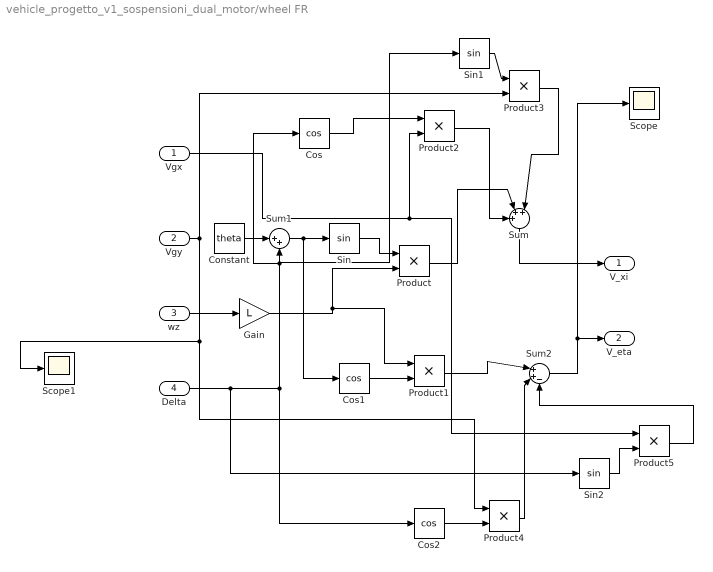
== system vehicle_progetto_v1_sospensioni_dual_motor/wheel FR ==
  Vgx : Inport
  Vgy : Inport  Port=2
  wz : Inport  Port=3
  Delta : Inport  Port=4
  Constant : Constant  Value=theta
  Cos : Trigonometry  Operator=cos
  Cos1 : Trigonometry  Operator=cos
  Cos2 : Trigonometry  Operator=cos
  Gain : Gain  Gain=L
  Product{,1..5} (6 alike) : Product
  Scope : Scope
  Scope1 : Scope
  Sin : Trigonometry
  Sin1 : Trigonometry
  Sin2 : Trigonometry
  Sum : Sum  Inputs=+++|
  Sum1 : Sum  Inputs=|++
  Sum2 : Sum  Inputs=|++-
  V_xi : Outport
  V_eta : Outport  Port=2
  wires:
  Vgx/1 -> Product5/1, Product2/2
  wz/1 -> Gain/1
  Sin/1 -> Product/1
  Constant/1 -> Sum1/1
  Sum1/1 -> Cos1/1, Sin/1
  Delta/1 -> Sin2/1, Cos2/1, Cos/1, Sum1/2, Sin1/1
  Product/1 -> Sum/2
  Sum/1 -> V_xi/1
  Cos1/1 -> Product1/2
  Gain/1 -> Product/2, Product1/1
  Product1/1 -> Sum2/1
  Sum2/1 -> Scope/1, V_eta/1
  Vgy/1 -> Product4/1, Scope1/1, Product3/2
  Cos/1 -> Product2/1
  Product2/1 -> Sum/1
  Sin1/1 -> Product3/1
  Product3/1 -> Sum/3
  Cos2/1 -> Product4/2
  Product4/1 -> Sum2/2
  Sin2/1 -> Product5/2
  Product5/1 -> Sum2/3

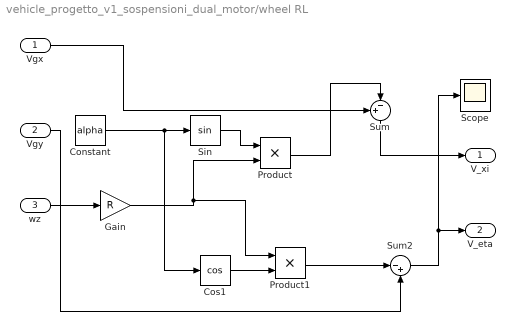
== system vehicle_progetto_v1_sospensioni_dual_motor/wheel RL ==
  Vgx : Inport
  Vgy : Inport  Port=2
  wz : Inport  Port=3
  Constant : Constant  Value=alpha
  Cos1 : Trigonometry  Operator=cos
  Gain : Gain  Gain=R
  Product : Product
  Product1 : Product
  Scope : Scope
  Sin : Trigonometry
  Sum : Sum  Inputs=+-|
  Sum2 : Sum  Inputs=|-+
  V_xi : Outport
  V_eta : Outport  Port=2
  wires:
  Vgx/1 -> Sum/1
  wz/1 -> Gain/1
  Sin/1 -> Product/1
  Constant/1 -> Cos1/1, Sin/1
  Product/1 -> Sum/2
  Sum/1 -> V_xi/1
  Cos1/1 -> Product1/2
  Gain/1 -> Product/2, Product1/1
  Product1/1 -> Sum2/1
  Sum2/1 -> Scope/1, V_eta/1
  Vgy/1 -> Sum2/2

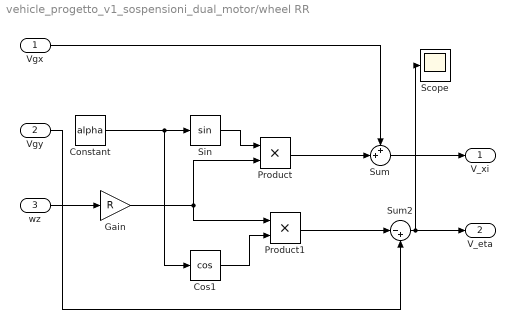
== system vehicle_progetto_v1_sospensioni_dual_motor/wheel RR ==
  Vgx : Inport
  Vgy : Inport  Port=2
  wz : Inport  Port=3
  Constant : Constant  Value=alpha
  Cos1 : Trigonometry  Operator=cos
  Gain : Gain  Gain=R
  Product : Product
  Product1 : Product
  Scope : Scope
  Sin : Trigonometry
  Sum : Sum  Inputs=++|
  Sum2 : Sum  Inputs=|-+
  V_xi : Outport
  V_eta : Outport  Port=2
  wires:
  Vgx/1 -> Sum/1
  wz/1 -> Gain/1
  Sin/1 -> Product/1
  Constant/1 -> Cos1/1, Sin/1
  Product/1 -> Sum/2
  Sum/1 -> V_xi/1
  Cos1/1 -> Product1/2
  Gain/1 -> Product/2, Product1/1
  Product1/1 -> Sum2/1
  Sum2/1 -> Scope/1, V_eta/1
  Vgy/1 -> Sum2/2

== matlab function vehicle_progetto_v1_sospensioni_dual_motor/tire RR/MATLAB Function ==
  data: Vc_xi input; y output; Fz input; w_y input; r parameter; mu_st parameter; k_r parameter; mu_dyn parameter; k_tv parameter; k_tu parameter; z output; Vc_eta input; delta output; gamma output
function [y,z,delta, gamma] = fcn(Vc_xi, Fz, w_y,r, mu_st, k_r, mu_dyn, k_tv, k_tu, Vc_eta)
c = (Fz*r*12/(k_r*0.2))^(1/3);
S = c*0.2;
sigma=(Vc_xi-w_y*r)/Vc_xi;
gamma = Vc_eta/Vc_xi;
delta = r*2*sqrt(k_tu^2*sigma^2+k_tv^2*gamma^2)/(c*mu_st*k_r);
if delta>1
    delta=1;
end
F_xi = -sign(Vc_xi-w_y*r)*mu_st*Fz*(6*abs(sigma)/(sqrt(sigma^2+gamma^2))*mu_dyn/mu_st*(0.5-1/3*delta)*(delta)^2+S*k_tu*c/(2*mu_st*Fz)*(delta-1)^2*abs(sigma));
F_eta = -sign(Vc_eta)*abs(mu_st*Fz*(6*gamma/(sqrt(sigma^2+gamma^2))*mu_dyn/mu_st*(0.5-1/3*delta)*(delta)^2+S*k_tv*c/(2*mu_st*Fz)*(delta-1)^2*gamma));
y = F_xi;
z = F_eta;

== matlab function vehicle_progetto_v1_sospensioni_dual_motor/tire FR/MATLAB Function ==
  data: Vc_xi input; y output; Fz input; w_y input; r parameter; mu_st parameter; k_r parameter; mu_dyn parameter; k_tv parameter; k_tu parameter; z output; Vc_eta input; delta output; gamma output
function [y,z, delta, gamma] = fcn(Vc_xi, Fz, w_y,r, mu_st, k_r, mu_dyn, k_tv, k_tu, Vc_eta)
c = (Fz*r*12/(k_r*0.2))^(1/3);
S = c*0.2;
sigma=(Vc_xi-w_y*r)/Vc_xi;
gamma = Vc_eta/Vc_xi;
delta = r*2*sqrt(k_tu^2*sigma^2+k_tv^2*gamma^2)/(c*mu_st*k_r);
if delta>1
    delta=1;
end
F_xi = -sign(Vc_xi-w_y*r)*mu_st*Fz*(6*abs(sigma)/(sqrt(sigma^2+gamma^2))*mu_dyn/mu_st*(0.5-1/3*delta)*(delta)^2+S*k_tu*c/(2*mu_st*Fz)*(delta-1)^2*abs(sigma));
F_eta = -sign(Vc_eta)*abs(mu_st*Fz*(6*gamma/(sqrt(sigma^2+gamma^2))*mu_dyn/mu_st*(0.5-1/3*delta)*(delta)^2+S*k_tv*c/(2*mu_st*Fz)*(delta-1)^2*gamma));
y = F_xi;
z = F_eta;

== matlab function vehicle_progetto_v1_sospensioni_dual_motor/Subsystem1/MATLAB Function ==
  data: delta input; w_kinematics output; vgx input; a parameter; b parameter
function w_kinematics = fcn(delta, vgx, a, b)
beta = atan(b*tan(delta)/(a+b));
w_kinematics = vgx*tan(delta)*cos(beta)/(a+b);

== matlab function vehicle_progetto_v1_sospensioni_dual_motor/Subsystem2/MATLAB Function ==
  data: u input; delta_sx output; delta_dx output; a parameter; b parameter; w parameter
function [delta_sx,delta_dx]= fcn(u, a, b, w)
delta_sx = atan(2*(a+b)*sin(u)/(2*(a+b)*cos(u)-w*sin(u)));
delta_dx = atan(2*(a+b)*sin(u)/(2*(a+b)*cos(u)+w*sin(u)));
y = u;

== matlab function vehicle_progetto_v1_sospensioni_dual_motor/Suspensions/FR susp ==
  data: phi input; f_FR output; beta input; Dphi input; Dbeta input; z input; Dz input; road input; Droad input; a parameter; b parameter; w parameter; cs parameter; ks parameter
function f_FR = fcn(phi, beta, Dphi, Dbeta, z, Dz, road, Droad, a, b, w, cs, ks)
%FR 
k_susp = ks;
c_susp = cs;
z_susp = z-a*sin(beta)-w/2*sin(phi);
Dz_susp = Dz-Dbeta*a*cos(beta)-Dphi*w/2*cos(phi);
if z_susp-road>0
    k_susp = 0;
    c_susp = 0;
end
f_FR = -k_susp*(z_susp-road)-c_susp*(Dz_susp-Droad);

== matlab function vehicle_progetto_v1_sospensioni_dual_motor/Suspensions/RR susp ==
  data: phi input; f_RR output; beta input; Dphi input; Dbeta input; z input; Dz input; road input; Droad input; a parameter; b parameter; w parameter; cs parameter; ks parameter
function f_RR = fcn(phi, beta, Dphi, Dbeta, z, Dz, road, Droad, a, b, w, cs, ks)
%RR 
k_susp = ks;
c_susp = cs;
z_susp = z+b*sin(beta)-w/2*sin(phi);
Dz_susp = Dz+Dbeta*b*cos(beta)-Dphi*w/2*cos(phi);
if z_susp-road>0
    k_susp = 0;
    c_susp = 0;
end
f_RR = -k_susp*(z_susp-road)-c_susp*(Dz_susp-Droad);

== matlab function vehicle_progetto_v1_sospensioni_dual_motor/Suspensions/FL susp ==
  data: phi input; f_FL output; beta input; Dphi input; Dbeta input; z input; Dz input; road input; Droad input; a parameter; b parameter; w parameter; cs parameter; ks parameter
function f_FL = fcn(phi, beta, Dphi, Dbeta, z, Dz, road, Droad, a, b, w, cs, ks)
%FL 
k_susp = ks;
c_susp = cs;
z_susp = z-a*sin(beta)+w/2*sin(phi);
Dz_susp = Dz-Dbeta*a*cos(beta)+Dphi*w/2*cos(phi);
if z_susp-road>0
    k_susp = 0;
    c_susp = 0;
end
f_FL = -k_susp*(z_susp-road)-c_susp*(Dz_susp-Droad);

== matlab function vehicle_progetto_v1_sospensioni_dual_motor/Suspensions/RL susp ==
  data: phi input; f_RL output; beta input; Dphi input; Dbeta input; z input; Dz input; road input; Droad input; a parameter; b parameter; w parameter; cs parameter; ks parameter
function f_RL = fcn(phi, beta, Dphi, Dbeta, z, Dz, road, Droad, a, b, w, cs, ks)
%RL 
k_susp = ks;
c_susp = cs;
z_susp = z+b*sin(beta)+w/2*sin(phi);
Dz_susp = Dz+Dbeta*b*cos(beta)+Dphi*w/2*cos(phi);
if z_susp-road>0
    k_susp = 0;
    c_susp = 0;
end
f_RL = -k_susp*(z_susp-road)-c_susp*(Dz_susp-Droad);

== matlab function vehicle_progetto_v1_sospensioni_dual_motor/MATLAB Function ==
  data: gamma input; y output; delta input; a parameter; b parameter
function y = fcn(gamma, delta, a, b)
%rear
l= a+b;
R_r = sqrt((l^2*(1+gamma^2))/(-gamma+tan(delta))^2);
R_f = sqrt((l/(gamma-tan(delta))^2)+((gamma*l)/gamma-tan(delta)-l)^2)
y = (R_f*b+R_r*a)/(a+b);
%y = R_r;

== matlab function vehicle_progetto_v1_sospensioni_dual_motor/tire RL/MATLAB Function ==
  data: Vc_xi input; y output; Fz input; w_y input; r parameter; mu_st parameter; k_r parameter; mu_dyn parameter; k_tv parameter; k_tu parameter; z output; Vc_eta input
function [y,z] = fcn(Vc_xi, Fz, w_y,r, mu_st, k_r, mu_dyn, k_tv, k_tu, Vc_eta)
c = (Fz*r*12/(k_r*0.2))^(1/3);
S = c*0.2;
sigma=(Vc_xi-w_y*r)/Vc_xi;
gamma = Vc_eta/Vc_xi;
delta = r*2*sqrt(k_tu^2*sigma^2+k_tv^2*gamma^2)/(c*mu_st*k_r);
if delta>1
    delta=1;
end
F_xi = -sign(Vc_xi-w_y*r)*mu_st*Fz*(6*abs(sigma)/(sqrt(sigma^2+gamma^2))*mu_dyn/mu_st*(0.5-1/3*delta)*(delta)^2+S*k_tu*c/(2*mu_st*Fz)*(delta-1)^2*abs(sigma));
F_eta = -sign(Vc_eta)*abs(mu_st*Fz*(6*gamma/(sqrt(sigma^2+gamma^2))*mu_dyn/mu_st*(0.5-1/3*delta)*(delta)^2+S*k_tv*c/(2*mu_st*Fz)*(delta-1)^2*gamma));
y = F_xi;
z = F_eta;

== matlab function vehicle_progetto_v1_sospensioni_dual_motor/tire FL/MATLAB Function ==
  data: Vc_xi input; y output; Fz input; w_y input; r parameter; mu_st parameter; k_r parameter; mu_dyn parameter; k_tv parameter; k_tu parameter; z output; Vc_eta input; sigma output; gamma output; delta output
function [y,z,sigma,gamma,delta] = fcn(Vc_xi, Fz, w_y,r, mu_st, k_r, mu_dyn, k_tv, k_tu, Vc_eta)
c = (Fz*r*12/(k_r*0.2))^(1/3);
S = c*0.2;
sigma=(Vc_xi-w_y*r)/Vc_xi;
gamma = Vc_eta/Vc_xi;
delta = r*2*sqrt(k_tu^2*sigma^2+k_tv^2*gamma^2)/(c*mu_st*k_r);
if delta>1
    delta=1;
end
F_xi = -sign(Vc_xi-w_y*r)*mu_st*Fz*(6*abs(sigma)/(sqrt(sigma^2+gamma^2))*mu_dyn/mu_st*(0.5-1/3*delta)*(delta)^2+S*k_tu*c/(2*mu_st*Fz)*(delta-1)^2*abs(sigma));
F_eta = -sign(Vc_eta)*abs(mu_st*Fz*(6*gamma/(sqrt(sigma^2+gamma^2))*mu_dyn/mu_st*(0.5-1/3*delta)*(delta)^2+S*k_tv*c/(2*mu_st*Fz)*(delta-1)^2*gamma));
y = F_xi;
z = F_eta;

== matlab function vehicle_progetto_v1_sospensioni_dual_motor/Subsystem/MATLAB Function ==
  data: Vgy input; Vgy_dot output; wz input; Vgx input; delta input; F_xi_FL input; F_eta_FL input; F_xi_FR input; F_eta_FR input; F_xi_RL input; F_eta_RL input; F_xi_RR input; F_eta_RR input; M parameter; a parameter; b parameter; h_gc parameter; Jx parameter; Jy parameter; Jz parameter; ca parameter; FL input; FR input; RR input; RL input; wz_dot output; Vgx_dot output; phi_dot_dot output; beta_dot_dot output; w parameter
function [Vgy_dot, wz_dot, Vgx_dot, phi_dot_dot, beta_dot_dot] = fcn(Vgy, wz, Vgx, delta, F_xi_FL, F_eta_FL,  F_xi_FR, F_eta_FR,  F_xi_RL, F_eta_RL, F_xi_RR, F_eta_RR, M, a, b, h_gc, Jx, Jy, Jz, ca, FL, FR, RR, RL, w )

F_air=ca*Vgx^2;
Fy = (F_eta_RL + F_eta_RR)+ (F_eta_FL + F_eta_FR)*cos(delta) + (F_xi_FL + F_xi_FR)*sin(delta); %data dalla trazione delle ruote

% disp(F_eta_RL)
% disp(F_eta_RR)
% disp(F_eta_FR)
% disp(F_xi_FL)
% disp(F_xi_FR)
% disp(Fy)
% disp(M)
% disp(wz)
% disp(Vgx)

Vgy_dot = Fy/M - wz*Vgx ;
% disp(Vgy_dot)

Mgz = -(F_eta_RL + F_eta_RR)*b+(F_eta_FL + F_eta_FR)*cos(delta)*a+(F_xi_FL + F_xi_FR)*sin(delta)*a;
wz_dot = Mgz/Jz;
Fx = (F_xi_RL + F_xi_RR)+(F_xi_FL + F_xi_FR)*cos(delta)-(F_eta_FL + F_eta_FR)*sin(delta);
Vgx_dot = Fx/M -F_air/M*sign(Vgx);
phi_dot_dot = 1/Jx*(FL+RL-FR-RR)*w/2 + Fy*h_gc/Jx;
My = Fx*h_gc;
beta_dot_dot = 1/Jy*(RR+RL)*b - 1/Jy*(FL+FR)*a - My/Jy;
